simulink model "porownanie_antek"  (R2019a)
settings: Solver=VariableStepAuto  StartTime=0.0  StopTime=1000  RelTol=1e-3
libraries: simulink x1
settings Model: Creator=hpiet  LastModifiedBy=hpiet
settings DebuggingCC: UnconnectedInputMsg=none  UnconnectedOutputMsg=none  UnconnectedLineMsg=none  SFMachineParentedDataDiag=error
settings ModelReferenceCC: EnableRefExpFcnMdlSchedulingChecks=off
settings RTWCC: Description=Generic Real-Time Target

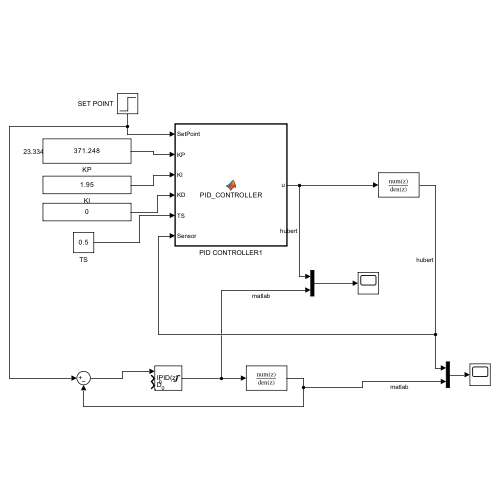
[thumbnail: Simulink's stored preview of the top-level diagram]
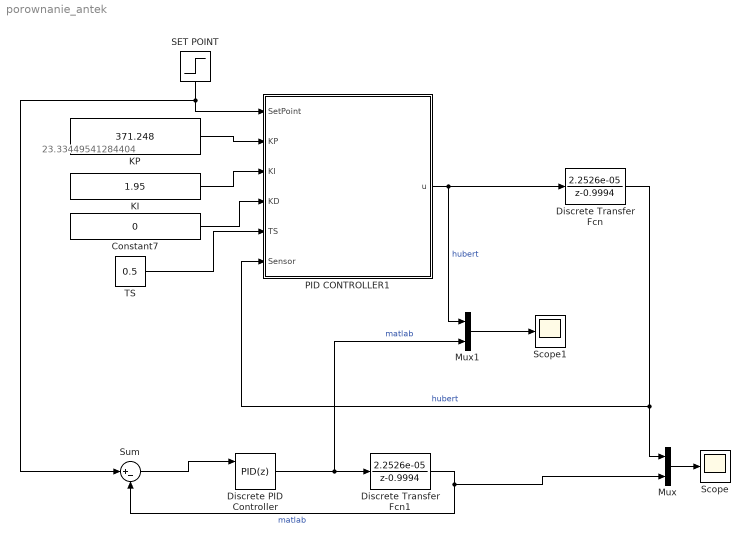
== system porownanie_antek ==
  note: 23.33449541284404
  Constant7 : Constant  Value=0
  Discrete Transfer Fcn : DiscreteTransferFcn  Numerator=[2.2526e-05]  Denominator=[1 -0.9994]  SampleTime=0.5
  Discrete Transfer Fcn1 : DiscreteTransferFcn  Numerator=[2.2526e-05]  Denominator=[1 -0.9994]
  Discrete PID Controller : simulink/Continuous/PID Controller  Controller=PID  Form=Parallel  TimeDomain=Discrete-time  SampleTime=0.5  IntegratorMethod=Forward Euler  ControllerParametersSource=internal  P=371.248  I=1.95  D=0  N=0.03  UseFilter=on  TunerSelectOption=Transfer Function Based (PID Tuner App)  InitialConditionSource=external  InitialConditionForIntegrator=0  InitialConditionForFilter=0  DifferentiatorICPrevScaledInput=0  ExternalReset=none  TrackingMode=off  Kt=1  LimitOutput=on  UpperSaturationLimit=100  LowerSaturationLimit=0  LinearizeAsGain=off  AntiWindupMode=none  Kb=0.1  POutMin=[]  POutMax=[]  IOutMin=[]  IOutMax=[]  DOutMin=[]  DOutMax=[]  NOutMin=[]  NOutMax=[]  SumOutMin=[]  SumOutMax=[]  SaturationOutMin=[]  SaturationOutMax=[]  PParamMin=[]  PParamMax=[]  IParamMin=[]  IParamMax=[]  DParamMin=[]  DParamMax=[]  NParamMin=[]  NParamMax=[]  KbParamMin=[]  KbParamMax=[]  KtParamMin=[]  KtParamMax=[]  KbOutMin=[]  KbOutMax=[]  KtOutMin=[]  KtOutMax=[]  IntegratorOutMin=[]  IntegratorOutMax=[]  FilterOutMin=[]  FilterOutMax=[]  SumI1OutMin=[]  SumI1OutMax=[]  SumI2OutMin=[]  SumI2OutMax=[]  SumI3OutMin=[]  SumI3OutMax=[]  SumI4OutMin=[]  SumI4OutMax=[]  SumDOutMin=[]  SumDOutMax=[]  DifferentiatorOutMin=[]  DifferentiatorOutMax=[]  FilterDiffOutCoefMin=[]  FilterDiffOutCoefMax=[]  ReciprocalOutMin=[]  ReciprocalOutMax=[]  SumDenOutMin=[]  SumDenOutMax=[]  SumNumOutMin=[]  SumNumOutMax=[]  DivideOutMin=[]  DivideOutMax=[]  IntegratorContinuousStateAttributes=''  IntegratorStateMustResolveToSignalObject=off  IntegratorRTWStateStorageClass=Auto  FilterContinuousStateAttributes=''  FilterStateMustResolveToSignalObject=off  FilterRTWStateStorageClass=Auto  ParallelPVariant=InternalParameters  IdealPVariant=Disabled  IVariant=InternalParameters  DVariant=InternalParameters  IntegratorVariant=Discrete  SatVariant=Enabled  AWVariant=Passthrough  PCopyVariant=Disabled  TRVariant=Disabled  FdbkBlocksVariant=Forward  IdealPFdbkVariant=Disabled  SatFdbkVariant=Disabled  DerivativeFilterVariant=ForwardEulerFilter  NVariant=InternalParameters  NCopyVariant=Disabled  FilterICVariant=ExternalICs  IntegratorICVariant=ExternalICs  ExternalResetVariant=Disabled  TRSumVariant=Passthrough  SumFdbkVariant=Disabled  SumVariant=Sum_PID
  KI : Constant  Value=1.95
  KP : Constant  Value=371.248
  Mux : Mux  Inputs=2
  Mux1 : Mux  Inputs=2
  PID CONTROLLER1 : MATLAB Function  TreatAsAtomicUnit=on
  SET POINT : Step  Time=0  SampleTime=0.5
  Scope : Scope
  Scope1 : Scope
  Sum : Sum  Inputs=|+-
  TS : Constant  Value=0.5  VectorParams1D=off
  wires:
  TS/1 -> PID CONTROLLER1/5(TS)
  KI/1 -> PID CONTROLLER1/3(KI)
  Discrete Transfer Fcn/1 -> Mux/1, PID CONTROLLER1/6(Sensor)  "hubert"
  SET POINT/1 -> Sum/1, PID CONTROLLER1/1(SetPoint)
  KP/1 -> PID CONTROLLER1/2(KP)
  Constant7/1 -> PID CONTROLLER1/4(KD)
  PID CONTROLLER1/1(u) -> Discrete Transfer Fcn/1, Mux1/1  "hubert"
  Sum/1 -> Discrete PID Controller/1
  Discrete PID Controller/1 -> Mux1/2, Discrete Transfer Fcn1/1  "matlab"
  Discrete Transfer Fcn1/1 -> Mux/2, Sum/2  "matlab"
  Mux/1 -> Scope/1
  Mux1/1 -> Scope1/1

== matlab function porownanie_antek/PID CONTROLLER1 ==
  settings: updateMethod=DISCRETE
  data: SetPoint input; KP input; KI input; KD input; TS input; u output; Sensor input
function u = PID_CONTROLLER(SetPoint, KP, KI, KD, TS, Sensor) 

persistent init u1 u2 e1 e2 KU1 KU2 KE0 KE1 KE2 integral_error sat_upper sat_lower Kfi after_sat_signal;

if isempty(init)
%INICJALIZACJA FUNKCJI Z SKRYPTU MATLAB
[KU1,KU2,KE0,KE1,KE2]=PID_init(KP,KI,KD,TS);
e2=0;
e1=0;
u2=0;
u1=0;
sat_upper = 100;
sat_lower= 0;


after_sat_signal=0;
Kfi=1;
integral_error=0;

init=1;
end

%Definicja uchybu i równanie sterowania PID
e0=SetPoint-Sensor;


u0 = -KU1*u1 - (KU2 * u2) + (KE0*e0) + (KE1*e1) + (KE2*e2)+integral_error;
% if(u0<=sat_upper && u0=>sat_lower)
%    integral_error = Kfi*(after_sat_signal-u0);
%     elseif(u0 > sat_upper) 
%         integral_error =  Kfi*(after_sat_signal-u0);
%     elseif ( u0 < sat_lower)
%         integral_error =  Kfi*(after_sat_signal-u0);
% end
if(integral_error==0)
    disp('intergral 0')
end
e2=e1;
e1=e0;
u2=u1;
u1=u0;

if(u0 > sat_upper) 
    after_sat_signal= sat_upper;
elseif ( u0 < sat_lower)
    after_sat_signal= sat_lower;     %do innej zmiennej v
else
    after_sat_signal=u0;
end


u=u0;
end





%BZDURY
% integral_error=integral_error + KE0*e0;
% presat_integral_error = integral_error;
% PD=(KE1*e1) + (KE2*e2);
% 
% u0 = -(KU1*u1) - (KU2 * u2) + (KE0*e0) + (KE1*e1) + (KE2*e2);
% 
% %ANTY WINDUP
% 
% if(u0 > sat_upper)
%     u0= sat_upper;
% elseif ( u0 < sat_lower)
%     u0= sat_lower;
% end
% 
% 
% integral_error = presat_integral_error + (u0 - (PD))/(KE0);
% 
% e2=e1;
% e1=e0;
% u2=u1;
% u1=u0;
% 
% u=u0;
% 
% end
